simulink model "auditory_nerve"  (R2020b)
settings: Solver=FixedStepDiscrete  StartTime=0.0  StopTime=stopTime  FixedStep=2.0833333333333333e-05  RelTol=1e-3
InitFcn:
  | initCallback
StopFcn:
  | stopCallback
undefined symbols (not defined in the file or in its folder): mp, rsigma
settings Model: Creator=Ross  LastModifiedBy=conno
settings DataIOCC: SaveOutput=off  SaveTime=off  ReturnWorkspaceOutputs=off
settings OptimizationCC: BlockReduction=off  ConditionallyExecuteInputs=off  DefaultParameterBehavior=Inlined
settings DebuggingCC: ReadBeforeWriteMsg=DisableAll  WriteAfterWriteMsg=DisableAll  WriteAfterReadMsg=DisableAll  AlgebraicLoopMsg=error  MultiTaskDSMMsg=none  SingleTaskRateTransMsg=error  PregeneratedLibrarySubsystemCodeDiagnostic=none  ArithmeticOperatorsInVariantConditions=warning
settings HardwareCC: ProdBitPerPointer=32  ProdBitPerSizeT=32  ProdBitPerPtrDiffT=32  ProdLargestAtomicFloat=None  ProdIntDivRoundTo=Undefined  ProdEndianess=Unspecified  ProdWordSize=32  ProdHWDeviceType=ASIC/FPGA->ASIC/FPGA  TargetBitPerPointer=64  TargetBitPerSizeT=64  TargetBitPerPtrDiffT=64  TargetLongLongMode=on  TargetIntDivRoundTo=Zero  TargetEndianess=LittleEndian  TargetWordSize=64  TargetHWDeviceType=Custom Processor->MATLAB Host Computer  ProdEqTarget=off
settings ModelReferenceCC: UpdateModelReferenceTargets=IfOutOfDate
settings SFSimCC: SFSimEcho=off  SimUseLocalCustomCode=off  CustomCodeUndefinedFunction=UseInterfaceOnly
settings RTWCC: RTWUseLocalCustomCode=off

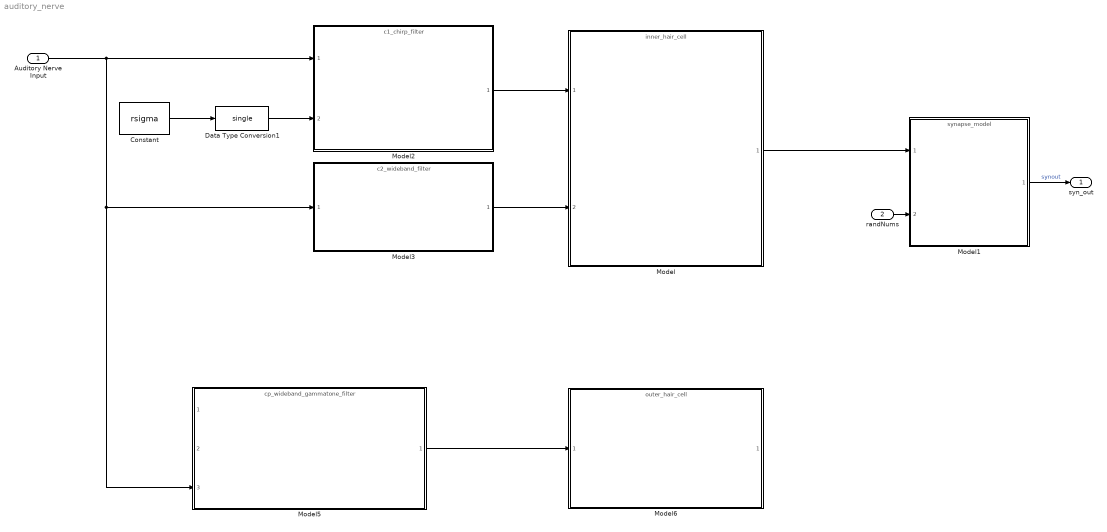
== system auditory_nerve ==
  Auditory Nerve Input : Inport  OutDataTypeStr=single  PortDimensions=1  SampleTime=[2.0833333333333333e-05,0]
  randNums : Inport  Port=2  OutDataTypeStr=single  PortDimensions=[1 1]  SampleTime=[2.0833333333333333e-05,0]
  Constant : Constant  Value=rsigma  SampleTime=mp.Ts_sim
  Data Type Conversion1 : DataTypeConversion  OutDataTypeStr=single  RndMeth=Nearest
  Model : ModelReference  ModelNameDialog=inner_hair_cell.slx  SimulationMode=Normal  ModelReferenceVersion=1.135
  Model1 : ModelReference  ModelNameDialog=synapse_model.slx  SimulationMode=Normal  ModelReferenceVersion=1.137
  Model2 : ModelReference  ModelNameDialog=c1_chirp_filter.slx  SimulationMode=Normal  ModelReferenceVersion=1.120
  Model3 : ModelReference  ModelNameDialog=c2_wideband_filter.slx  SimulationMode=Normal  ModelReferenceVersion=1.111
  Model5 : ModelReference  ModelNameDialog=cp_wideband_gammatone_filter.slx  SimulationMode=Normal  ModelReferenceVersion=1.112
  Model6 : ModelReference  ModelNameDialog=outer_hair_cell.slx  SimulationMode=Normal  ModelReferenceVersion=1.125
  syn_out : Outport  OutDataTypeStr=single  PortDimensions=1  SampleTime=[2.0833333333333333e-05,0]  InitialOutput=0  VectorParamsAs1DForOutWhenUnconnected=off
  wires:
  Model3/1 -> Model/2
  Model1/1 -> syn_out/1  "synout"
  Model/1 -> Model1/1
  Model2/1 -> Model/1
  randNums/1 -> Model1/2
  Data Type Conversion1/1 -> Model2/2
  Constant/1 -> Data Type Conversion1/1
  Auditory Nerve Input/1 -> Model2/1, Model5/3, Model3/1
  Model5/1 -> Model6/1
